simulink model "IndustrialMicrogrid"  (R2025a)
settings: Solver=FixedStepAuto  StartTime=0.0  StopTime=8  FixedStep=Ts  RelTol=1e-3
PostLoadFcn:
  | IndustrialMicrogridInputData
  | GfmGridFormingConverterInputParameters
model workspace (MAT data in the model file):
  caseNum = 2
undefined symbols (not defined in the file): base, BESS, DiscIntNeverNeededParam, grid, Grid, gridInverter, machine, microgrid, PV, PVInverter, PVTransformer, scrFactorRg, scrFactorXg, transformer, Transition_and_Dispatch_ControlModeType, Ts
libraries: ee_lib x126, fl_lib x91, eeGeneralControl x73, nesl_utility x50, nesl_utility_internal x46, simulink x30, eeTransforms x11, eeSinusoidalMeasurementV2 x5, eeTotalHarmonicDistorsion x4, slpidlib x3, simulink_extras x2, eePowerMeasurement x2
(part 12 of 12)

== stateflow chart IndustrialMicrogrid/MG1 Primary Substation/Microgrid Controller/Microgrid Supervisory Control/Transition and Dispatch Control ==
  state On
    entry:
    BrKControl.PCC = BreakerStatus;
    resyncDispatch = false;
    plannedIslandingDispatch = false;
    emergencyDispatch = false;
    state Steady_State_Islanded
    state Steady_State_Grid_Connected
    state Resynchronization
    state Unplanned_Islanding
    state Black_Start
    state Planned_Islanding
    (default) -> (junction 282)
    (junction 403) -> Steady_State_Islanded
    (junction 401) -> (junction 403)
    Steady_State_Grid_Connected -> (junction 317) : [PlannedIslanding.enable == true &&...
        |  BreakerStatus <=0]
    (junction 282) -> Steady_State_Grid_Connected [order 2] : [BreakerStatus <= 0 && ...
        | PlannedIslanding.enable == false...
        | && BlackStart.blackout == false]
    (junction 282) -> Steady_State_Islanded [order 1] : [BreakerStatus > 0 && ...
        | Resync.enable == false && ...
        | BlackStart.blackout == false]
    (junction 317) -> (junction 338)
    (junction 282) -> (junction 312) [order 3]
    Steady_State_Islanded -> (junction 314) : [Resync.enable == true && ...
        | BreakerStatus > 0]
    (junction 314) -> (junction 329)
    Resynchronization -> Steady_State_Grid_Connected : [BreakerStatus <= 0 && ...
        | (Island.voltage > lowerVoltageLimit && ...
        | Island.voltage < upperVoltageLimit) && ...
        | (Island.frequency > lowerFrequencyLimit  && ...
        | Island.frequency  <  upperFrequencyLimit)]
    (junction 299) -> Steady_State_Islanded
    (junction 306) -> (junction 299)
    (junction 326) -> Resynchronization
    (junction 330) -> (junction 326)
    Unplanned_Islanding -> (junction 306) : [BreakerStatus > 0 && ...
        | (Island.voltage > lowerVoltageLimit && ...
        | Island.voltage < upperVoltageLimit) && ...
        | (Island.frequency > lowerFrequencyLimit  && ...
        | Island.frequency  <  upperFrequencyLimit)]
    (junction 312) -> Unplanned_Islanding [order 3]
    (junction 312) -> Resynchronization [order 1] : [Resync.enable == true && ...
        | BreakerStatus > 0]
    (junction 312) -> (junction 297) [order 2]
    (junction 285) -> (junction 306)
    On -> Unplanned_Islanding : [UnplannedIslandingEnable  > 0 && emergencyDispatch == false]
    (junction 297) -> Planned_Islanding [order 1] : [PlannedIslanding.enable == true &&...
        | BreakerStatus <= 0 ]
    (junction 297) -> Black_Start [order 2] : [BlackStart.blackout == true && ...
        | BreakerStatus >= 0]
    Planned_Islanding -> (junction 285) : [BreakerStatus > 0 && ...
        | (Island.voltage > lowerVoltageLimit && ...
        | Island.voltage < upperVoltageLimit) && ...
        | (Island.frequency > lowerFrequencyLimit  && ...
        | Island.frequency  <  upperFrequencyLimit)]
    Black_Start -> (junction 398)
    (junction 341) -> Planned_Islanding
    (junction 329) -> (junction 330)
    (junction 338) -> (junction 341)
    (junction 398) -> (junction 401) : [[ BlackStart.status == true  &&...
        | (Island.voltage > lowerVoltageLimit && ...
        | Island.voltage < upperVoltageLimit) && ...
        | (Island.frequency > lowerFrequencyLimit  && ...
        | Island.frequency  <  upperFrequencyLimit)]]
  (default) -> On
  data: plannedIslandingDispatch function_input; emergencyDispatch function_output; resyncDispatch function_input; emergencyDispatch function_output; PCC function_output; resync function_output; resyncStatus function_output; resyncDispatch function_output; PCC function_output; emergencyDispatch function_output; blackStartStatus function_output; blackStartComplete function_input; blackStart function_output; blackStartEnable function_input; PCC function_output; plannedIslanding function_output; plannedIslandingDispatch function_output; plannedIslandingStatus function_output; Resync input Bus: Resync; UnplannedIslandingEnable input; Island input Bus: Island; lowerVoltageLimit parameter; upperFrequencyLimit parameter; upperVoltageLimit parameter; BrKControl output Bus: BrKControl; Status output Bus: Status; BreakerStatus input; PlannedIslanding input Bus: PlannedIslanding; lowerFrequencyLimit parameter; resyncDispatch local boolean size=1; plannedIslandingDispatch local boolean size=1; emergencyDispatch local boolean size=1; BlackStart input Bus: BlackStart; Transition_and_Dispatch_ControlMode output Enum: Transition_and_Dispatch_ControlModeType

== stateflow chart IndustrialMicrogrid/MG1 Primary Substation/Microgrid Controller/Microgrid Supervisory Control/Transition and Dispatch Control/On.Black_Start ==
  state Entry
  state Enable
    blackStart = true;
  state Status
    blackStartStatus = true;
  (default) -> Entry
  Entry -> Enable : [blackStartEnable == true]
  Enable -> Status : [blackStartComplete == true]
  data: blackStartComplete input boolean; blackStartStatus output boolean; blackStart output boolean; blackStartEnable input

== stateflow chart IndustrialMicrogrid/MG2 Primary Substation/Microgrid Controller/Microgrid Supervisory Control/Transition and Dispatch Control/On.Resynchronization ==
  state Enable
    resync = true;
  state PCCBreakerClose
    resyncStatus = true;
    PCC = 0;
    resyncDispatch = true;
  (default) -> Enable
  Enable -> PCCBreakerClose : after(Resync.delay,sec)[Resync.status == true]
  data: Resync input Bus: Resync; PCC output double; resync output boolean; resyncStatus output boolean; resyncDispatch output boolean size=1

== stateflow chart IndustrialMicrogrid/MG2 Primary Substation/Microgrid Controller/Microgrid Supervisory Control/Transition and Dispatch Control/On.Steady_State_Grid_Connected ==
  state Steady_State
    emergencyDispatch = false;
  state Resync_actions
  (default) -> Steady_State
  Steady_State -> Resync_actions : after(0.2,sec)[resyncDispatch == true]
  data: emergencyDispatch output boolean; resyncDispatch input boolean size=1

== stateflow chart IndustrialMicrogrid/MG2 Primary Substation/Microgrid Controller/Microgrid Supervisory Control/Transition and Dispatch Control/On.Steady_State_Islanded ==
  state Steady_state
    emergencyDispatch = false;
  state BreakerControl
  (default) -> Steady_state
  Steady_state -> BreakerControl : after(0.5,sec)[plannedIslandingDispatch == true]
  data: plannedIslandingDispatch input boolean; emergencyDispatch output boolean

== stateflow chart IndustrialMicrogrid/MG2 Primary Substation/Microgrid Controller/Microgrid Supervisory Control/Transition and Dispatch Control/On.Unplanned_Islanding ==
  state TimeDelay
    emergencyDispatch = true;
  state BreakerEnable
    PCC = 1;
  (default) -> TimeDelay
  TimeDelay -> BreakerEnable : after(0.05,sec)
  data: PCC output double; emergencyDispatch output boolean

== stateflow chart IndustrialMicrogrid/MG2 Primary Substation/Microgrid Controller/Microgrid Supervisory Control/Transition and Dispatch Control/On.Black_Start ==
  state Entry
  state Enable
    blackStart = true;
  state Status
    blackStartStatus = true;
  (default) -> Entry
  Entry -> Enable : [blackStartEnable == true]
  Enable -> Status : [blackStartComplete == true]
  data: blackStartComplete input boolean; blackStartStatus output boolean; blackStart output boolean; blackStartEnable input

== stateflow chart IndustrialMicrogrid/MG1 Primary Substation/BESS and Controller/BESS/Grid-Forming Converter Control/Current Limiting/CurrentLimitingMethod/currentLimitAndVirtual/CurrentLimitSelection ==
  state Mode1_VI_ON
    entry:
    noCurrentLimit  = 0;
    viCurrentLimit = 1;
    satCurrentLimit = 0;
    ismax= maxVICurrentLimit;
    exit:
    noCurrentLimit  = 0;
    viCurrentLimit = 1;
    satCurrentLimit = 0;
    ismax= maxVICurrentLimit;
  state Start_Mode
    entry:
    noCurrentLimit  = 1;
    viCurrentLimit = 0;
    satCurrentLimit = 0;
    ismax= maxSatCurrentLimit;
    exit:
    noCurrentLimit  = 1;
    viCurrentLimit = 0;
    satCurrentLimit = 0;
    ismax= maxSatCurrentLimit;
  state Mode2_CurrentSat_ON
    entry:
    noCurrentLimit  = 0;
    viCurrentLimit = 0;
    satCurrentLimit = 1;
    ismax= maxSatCurrentLimit;
    exit:
    noCurrentLimit  = 0;
    viCurrentLimit = 0;
    satCurrentLimit = 1;
    ismax= maxSatCurrentLimit;
  state Mode3_CurrentSat_ON
    entry:
    noCurrentLimit  = 0;
    viCurrentLimit = 0;
    satCurrentLimit = 1;
    ismax= 1.1*maxVICurrentLimit;
    exit:
    noCurrentLimit  = 0;
    viCurrentLimit = 0;
    satCurrentLimit = 1;
    ismax= 1.1*maxVICurrentLimit;
  Start_Mode -> Mode1_VI_ON : [Is>1]
  (junction 28) -> Mode1_VI_ON : after(currentControlTs*10, sec)[(Is<ismax) && (Is>1) ]
  Mode3_CurrentSat_ON -> (junction 28) [order 1]
  (default) -> Start_Mode
  Mode1_VI_ON -> Start_Mode [order 2] : [Is<1]
  Mode1_VI_ON -> Mode2_CurrentSat_ON [order 1] : after(0.5/powerFreq, sec)[(Is>=maxSatCurrentLimit)]
  (junction 26) -> Start_Mode
  Mode3_CurrentSat_ON -> Mode2_CurrentSat_ON [order 2] : after(0.5/powerFreq, sec)[(Is>ismax)]
  Mode2_CurrentSat_ON -> Mode3_CurrentSat_ON : after(currentSatTime, sec)[satCurrentLimit>0]
  Mode3_CurrentSat_ON -> (junction 26) [order 3] : [Is<1]
  data: Is input; ismax output; noCurrentLimit output; viCurrentLimit output; satCurrentLimit output; maxSatCurrentLimit parameter; maxVICurrentLimit parameter; currentControlTs parameter; currentSatTime parameter; powerFreq parameter

== matlab function IndustrialMicrogrid/MG1 Primary Substation/BESS and Controller/BESS/Grid-Forming Converter Control/Measurement/Frequency Measurement/Frequency Measurement/If Action Subsystem/Frequency estimation/MATLAB Function ==
  data: y1 input; y2 input; x1 input; x output; x2 input
function x = fcn(y1,y2,x1,x2)
% Line equation between two points is y-y1=((y2-y1)/(x2-x1))*(x-x1). Here
% to to find the zero crossing instant substitute y = 0 and find x
slope = (y2-y1)/(x2-x1);
x = x1-y1/slope;

== stateflow chart IndustrialMicrogrid/MG1 Primary Substation/Microgrid Controller/Microgrid Supervisory Control/Transition and Dispatch Control/On.Planned_Islanding ==
  state Enable
    plannedIslanding = true;
  state BreakerOpen
    PCC = 1;
    plannedIslandingStatus = true;
    plannedIslandingDispatch = true;
  (default) -> Enable
  Enable -> BreakerOpen : after(PlannedIslanding.delay,sec)[PlannedIslanding.status == true]
  data: PlannedIslanding input Bus: PlannedIslanding; PCC output; plannedIslanding output boolean; plannedIslandingDispatch output boolean; plannedIslandingStatus output boolean

== stateflow chart IndustrialMicrogrid/MG1 Primary Substation/Microgrid Controller/Microgrid Supervisory Control/Transition and Dispatch Control/On.Resynchronization ==
  state Enable
    resync = true;
  state PCCBreakerClose
    resyncStatus = true;
    PCC = 0;
    resyncDispatch = true;
  (default) -> Enable
  Enable -> PCCBreakerClose : after(Resync.delay,sec)[Resync.status == true]
  data: Resync input Bus: Resync; PCC output double; resync output boolean; resyncStatus output boolean; resyncDispatch output boolean size=1

== stateflow chart IndustrialMicrogrid/MG1 Primary Substation/Microgrid Controller/Microgrid Supervisory Control/Transition and Dispatch Control/On.Steady_State_Grid_Connected ==
  state Steady_State
    emergencyDispatch = false;
  state Resync_actions
  (default) -> Steady_State
  Steady_State -> Resync_actions : after(0.2,sec)[resyncDispatch == true]
  data: emergencyDispatch output boolean; resyncDispatch input boolean size=1

== stateflow chart IndustrialMicrogrid/MG1 Primary Substation/Microgrid Controller/Microgrid Supervisory Control/Transition and Dispatch Control/On.Steady_State_Islanded ==
  state Steady_state
    emergencyDispatch = false;
  state BreakerControl
  (default) -> Steady_state
  Steady_state -> BreakerControl : after(0.5,sec)[plannedIslandingDispatch == true]
  data: plannedIslandingDispatch input boolean; emergencyDispatch output boolean

== stateflow chart IndustrialMicrogrid/MG1 Primary Substation/Microgrid Controller/Microgrid Supervisory Control/Transition and Dispatch Control/On.Unplanned_Islanding ==
  state TimeDelay
    emergencyDispatch = true;
  state BreakerEnable
    PCC = 1;
  (default) -> TimeDelay
  TimeDelay -> BreakerEnable : after(0.05,sec)
  data: PCC output double; emergencyDispatch output boolean
